simulink model "AttitudeComplementary"  (Simulink 6.6)
settings: Solver=ode4  StartTime=0.0  StopTime=300  FixedStep=SampleT  RelTol=1e-3
InitFcn:
  | clc
  | Taxi_Var_new
  | failures
  | insInit
values from neighbouring files (symbols this model uses):
  A1 = 0    [Taxi_Var.m]    (also in Taxi_Var_new.m = 0.007)
  Apolar = 0.0899    [Taxi_Var.m]    (also in Taxi_Var_new.m = 0.057)
  CD0 = 0.0219    [Taxi_Var.m]    (also in Taxi_Var_new.m = 0.022)
  chord = S/span    (= 0.384036716878)    [Taxi_Var.m]    (also in Taxi_Var_new.m = 0.351341681574)
  CL0 = 0.1857    [Taxi_Var.m]    (also in Taxi_Var_new.m = 0.38)
  CLa = 4.6206    [Taxi_Var.m]    (also in Taxi_Var_new.m = 18.5)
  CLa_dot = 1.93    [Taxi_Var.m]    (also in Taxi_Var_new.m = 2.64)
  Clb = -0.0043    [Taxi_Var.m]    (also in Taxi_Var_new.m = -0.06)
  ClDa = 0.1695    [Taxi_Var.m]    (also in Taxi_Var_new.m)
  CLDe = 0.4032    [Taxi_Var.m]    (also in Taxi_Var_new.m = 0.24)
  CLDf = 0.047    [Taxi_Var.m]    (also in Taxi_Var_new.m = 0.4)
  ClDr = 0.0003    [Taxi_Var.m]    (also in Taxi_Var_new.m = 0.055)
  Clp = -0.4425    [Taxi_Var.m]    (also in Taxi_Var_new.m = -0.88)
  CLq = 8.7465    [Taxi_Var.m]    (also in Taxi_Var_new.m = 7.4)
  Clr = 0.0675    [Taxi_Var.m]    (also in Taxi_Var_new.m = 0.04)
  Cm0 = -0.0902    [Taxi_Var.m]    (also in Taxi_Var_new.m = 0.56)
  Cma = -1.3995    [Taxi_Var.m]    (also in Taxi_Var_new.m = -1.58)
  CmDe = -0.9493    [Taxi_Var.m]    (also in Taxi_Var_new.m = -41)
  CmDf = -.021    (= -0.021)    [Taxi_Var.m]    (also in Taxi_Var_new.m)
  Cmq = -10.8760    (= -10.876)    [Taxi_Var.m]    (also in Taxi_Var_new.m = -12)
  Cnb = 0.0281    [Taxi_Var.m]    (also in Taxi_Var_new.m = 0.73)
  CnDa = -0.0031    [Taxi_Var.m]    (also in Taxi_Var_new.m = -0.032)
  CnDr = -0.0882    [Taxi_Var.m]    (also in Taxi_Var_new.m = 0.19)
  Cnp = -0.0695    [Taxi_Var.m]    (also in Taxi_Var_new.m = -0.1)
  Cnr = -0.1045    [Taxi_Var.m]    (also in Taxi_Var_new.m = -0.23)
  CYb = -0.1999    [Taxi_Var.m]    (also in Taxi_Var_new.m = -0.98)
  CYDr = 0.0192    [Taxi_Var.m]    (also in Taxi_Var_new.m = 0.066)
  Euler_0 = [0; 0; 45]'*pi/180    [Taxi_Var.m]    (also in Taxi_Var_new.m = [0 0 45]'*pi/180)
  ISA_g = 9.815    [Taxi_Var.m]    (also in Taxi_Var_new.m)
  Ixx = 3.689084    [Taxi_Var.m]    (also in Taxi_Var_new.m = 3.8)
  Iyy = 7.43789    [Taxi_Var.m]    (also in Taxi_Var_new.m = 9.58)
  Izz = 10.22202    [Taxi_Var.m]    (also in Taxi_Var_new.m = 9.68)
  mass = 22.5    [Taxi_Var.m]    (also in Taxi_Var_new.m = 8.16466266)
  MinThK = 0.075    [Taxi_Var.m]    (also in Taxi_Var_new.m = 0.077)
  Pos_0 = [0; 0; 1000]'    [Taxi_Var.m]    (also in Taxi_Var_new.m = [0 0 500]')
  PQR_0 = [0; 0; 0]'    [Taxi_Var.m]    (also in Taxi_Var_new.m = [ 0 0 0]'*pi/180)
  SampleT = 0.005    [failures.m]
  span = 2.3368    [Taxi_Var.m]    (also in Taxi_Var_new.m = 2.795)
  TFact = 0.4    [Taxi_Var.m]    (also in Taxi_Var_new.m)
  ThK = 2.18    [Taxi_Var.m]    (also in Taxi_Var_new.m = 2.17)
  Vb_0 = [35; 0; 0]'    [Taxi_Var.m]    (also in Taxi_Var_new.m = [35 0 0]')
undefined symbols (not defined in the file or in its folder): clock, DiscIntNeverNeededParam, Earth, gaind, polesd, sigbuilder_block, WGS84, zerosd
libraries: simulink x43, aerolibconvert2 x11, dspsigops x5, aerolibatmos2 x2, aerolibnav x2, dspmtrx3 x1, aerolibutil x1, aerolibtransform2 x1
(part 1 of 3)
CloseFcn:
  | rtwprivate ssgencode ModelCloseRequest AttitudeComplementary
settings Model: Creator=ASL_Lab  LastModifiedBy=ASL_Lab
settings DebuggingCC: MultiTaskDSMMsg=warning  MultiTaskCondExecSysMsg=none  StrictBusMsg=None
settings HardwareCC: TargetHWDeviceType=32-bit Generic
settings RTWCC: IncludeERTFirstTime=on

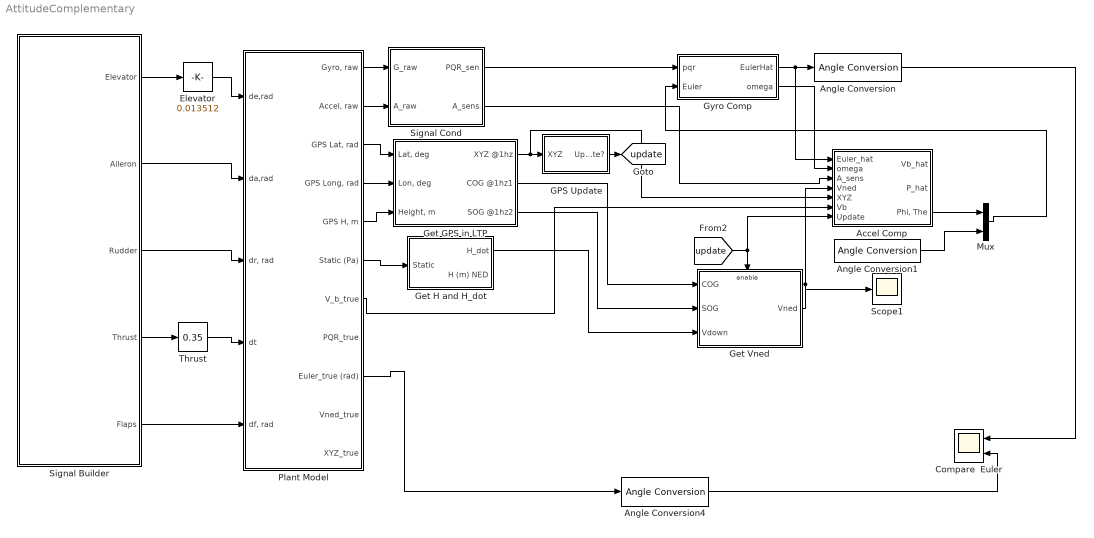
== system AttitudeComplementary ==
  Accel Comp : Subsystem
  Angle Conversion : aerolibconvert2/Angle Conversion  SystemSampleTime=-1  IU=rad  OU=deg
  Angle Conversion1 : aerolibconvert2/Angle Conversion  SystemSampleTime=-1  IU=deg  OU=rad
  Angle Conversion4 : aerolibconvert2/Angle Conversion  SystemSampleTime=-1  IU=rad  OU=deg
  Compare  Euler : Scope  NumInputPorts=2
      settings: TimeRange=150  YMin=-2.5~0  YMax=3.5~1.7  SaveName=ScopeData20
  Elevator : simulink/Math Operations/Slider Gain  SystemSampleTime=-1  low=-0.2  gain=0.013512  high=0.2
  GPS Update : Subsystem
  Get GPS in LTP : Subsystem
  "Get H and H_dot " : Subsystem
  Get Vned : Subsystem
  Gyro Comp : Subsystem
  Mux : Mux  Inputs=2
  Plant Model : Subsystem
  Scope1 : Scope
      settings: TimeRange=100  YMin=-60  YMax=80  SaveName=ScopeData27
  Signal Builder : Subsystem  Tag=STV Subsys  LoadFcn=sigbuilder_block('load');  StartFcn=sigbuilder_block('start');  StopFcn=sigbuilder_block('stop');  ClipboardFcn=sigbuilder_block('clipboard');  mask(Sigbuilder block){}
      mask help: Sigbuilder GUI
      mask init:
      | if ~strcmp(get_param(bdroot(gcbh),'SimulationStatus'),'stopped') tuvar = sigbuilder_block('maskInit'); end
      settings: CopyFcn=sigbuilder_block('copy');  DeleteFcn=sigbuilder_block('delete');  ModelCloseFcn=sigbuilder_block('modelClose');  PreSaveFcn=sigbuilder_block('preSave');  NameChangeFcn=sigbuilder_block('namechange');  OpenFcn=sigbuilder_block('open',[3 3 762 514.5 ]);  CloseFcn=sigbuilder_block('close');
      mask Display: plot(0,0,100,100,[10,10,40,40,10],[80,20,20,80,80],[40,10],[50,50], [40,27,10],[65,72,56],[40,25,25,10],[28,28,43,43]);
  Signal Cond : Subsystem
  Thrust : simulink/Math Operations/Slider Gain  SystemSampleTime=-1  low=0  gain=0.35  high=1
  tag scope: update=global
  wires:
  Signal Builder/4(Thrust) -> Thrust/1
  Thrust/1 -> Plant Model/4(dt)
  Signal Builder/1(Elevator) -> Elevator/1
  Signal Builder/2(Aileron) -> Plant Model/2(da,rad)
  Signal Builder/3(Rudder) -> Plant Model/3("dr, rad")
  Signal Builder/5(Flaps) -> Plant Model/5("df, rad")
  Elevator/1 -> Plant Model/1(de,rad)
  Plant Model/1("Gyro, raw") -> Signal Cond/1(G_raw)
  Plant Model/2("Accel, raw") -> Signal Cond/2(A_raw)
  Plant Model/3("GPS Lat, rad") -> Get GPS in LTP/1("Lat, deg")
  Plant Model/5("GPS H, m") -> Get GPS in LTP/3("Height, m")
  Plant Model/4("GPS Long, rad") -> Get GPS in LTP/2("Lon, deg")
  Signal Cond/2(A_sens) -> Accel Comp/3(A_sens)
  GPS Update/1(Update?) -> [update]
  Signal Cond/1(PQR_sen) -> Gyro Comp/1(pqr)
  [update] -> Get Vned/Enable, Accel Comp/7(Update)
  Gyro Comp/1(EulerHat) -> Angle Conversion/1, Accel Comp/1(Euler_hat)
  Angle Conversion/1 -> Compare  Euler/1
  Get Vned/1(Vned) -> Accel Comp/4(Vned), Scope1/1
  Accel Comp/3("Phi, The") -> Mux/1
  Angle Conversion1/1 -> Mux/2
  Mux/1 -> Gyro Comp/2(Euler)
  Plant Model/6(Static (Pa)) -> "Get H and H_dot "/1(Static)
  Get GPS in LTP/1(XYZ @1hz) -> GPS Update/1(XYZ), Accel Comp/5(XYZ)
  Gyro Comp/2(omega) -> Accel Comp/2(omega)
  Get GPS in LTP/2(COG @1hz1) -> Get Vned/1(COG)
  Get GPS in LTP/3(SOG @1hz2) -> Get Vned/2(SOG)
  "Get H and H_dot "/1(H_dot) -> Get Vned/3(Vdown)
  Plant Model/9(Euler_true (rad)) -> Angle Conversion4/1
  Plant Model/7(V_b_true) -> Accel Comp/6(Vb)
  Angle Conversion4/1 -> Compare  Euler/2

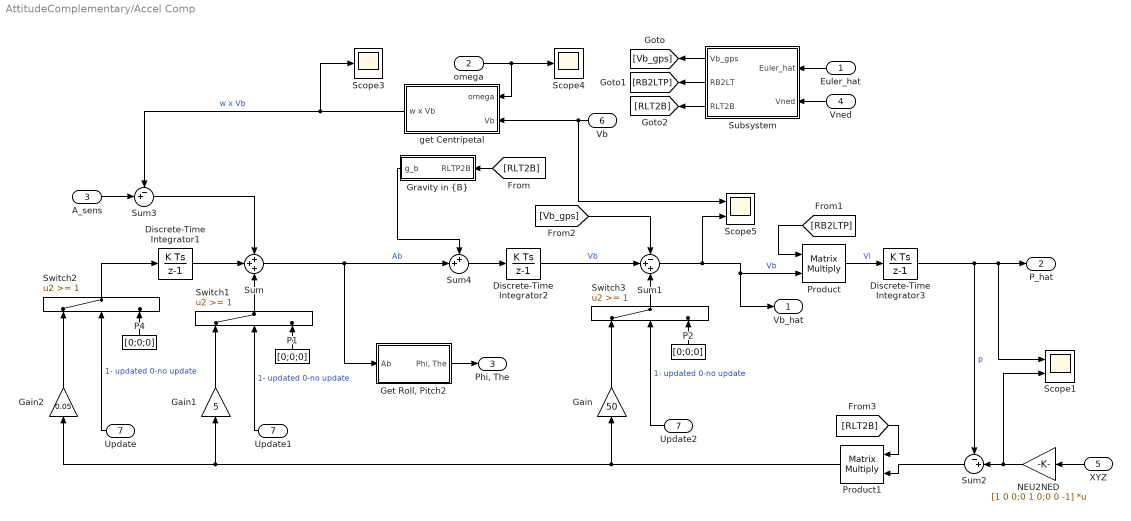
== system AttitudeComplementary/Accel Comp ==
  Euler_hat : Inport  Orientation=left
  omega : Inport  Port=2
  A_sens : Inport  Port=3
  Vned : Inport  Orientation=left  Port=4
  XYZ : Inport  Orientation=left  Port=5
  Vb : Inport  Orientation=left  Port=6
  Update : Inport  Orientation=left  Port=7
  Discrete-Time Integrator1 : DiscreteIntegrator  SampleTime=SampleT  ICPrevOutput=DiscIntNeverNeededParam  ICPrevScaledInput=DiscIntNeverNeededParam
  Discrete-Time Integrator2 : DiscreteIntegrator  InitialCondition=Vb_0  SampleTime=SampleT  ICPrevOutput=DiscIntNeverNeededParam  ICPrevScaledInput=DiscIntNeverNeededParam
  Discrete-Time Integrator3 : DiscreteIntegrator  InitialCondition=[Pos_0(1) Pos_0(2) -Pos_0(3)]  SampleTime=SampleT  ICPrevOutput=DiscIntNeverNeededParam  ICPrevScaledInput=DiscIntNeverNeededParam
  Gain : Gain  Orientation=up  Gain=50
  Gain1 : Gain  Orientation=up  Gain=5
  Gain2 : Gain  Orientation=up  Gain=0.05
  "Get Roll, Pitch2" : Subsystem
  "Gravity in {B}" : Subsystem  Orientation=left
  NEU2NED : Gain  Orientation=left  Gain=[1 0 0;0 1 0;0 0 -1]  Multiplication=Matrix(K*u)  SaturateOnIntegerOverflow=on
  P1 : Constant  Orientation=up  Value=[0;0;0]
  P2 : Constant  Orientation=up  Value=[0;0;0]
  P4 : Constant  Orientation=up  Value=[0;0;0]
  Product : Product  Multiplication=Matrix(*)  RndMeth=Zero
  Product1 : Product  Orientation=left  Multiplication=Matrix(*)  RndMeth=Zero
  Scope1 : Scope  NumInputPorts=2
      settings: TimeRange=300  YMin=-1500~-1500  YMax=8500~8500
  Scope3 : Scope
      settings: TimeRange=300  YMin=-10  YMax=4  SaveName=ScopeData26
  Scope4 : Scope
      settings: TimeRange=300  YMin=-0.1  YMax=0  SaveName=ScopeData29
  Scope5 : Scope  NumInputPorts=2
      settings: TimeRange=300  YMin=-2.5~-1750  YMax=35~3250  SaveName=ScopeData12
  Subsystem : Subsystem  Orientation=left
  Sum : Sum  Inputs=+++
  Sum1 : Sum  Inputs=-++
  Sum2 : Sum  Orientation=left  Inputs=-+|
  Sum3 : Sum  Inputs=-+|
  Sum4 : Sum  Inputs=++|
  Switch1 : Switch  Orientation=up  Threshold=1  SaturateOnIntegerOverflow=on
  Switch2 : Switch  Orientation=up  Threshold=1  SaturateOnIntegerOverflow=on
  Switch3 : Switch  Orientation=up  Threshold=1  SaturateOnIntegerOverflow=on
  Update1 : InportShadow  Orientation=left  Port=7  LatchByCopyingInsideSignal=off
  Update2 : InportShadow  Orientation=left  Port=7  LatchByCopyingInsideSignal=off
  get Centripetal : Subsystem  Orientation=left
  Vb_hat : Outport
  P_hat : Outport  Port=2
  "Phi, The" : Outport  Port=3
  wires:
  Sum2/1 -> Product1/2
  Discrete-Time Integrator3/1 -> Sum2/1, P_hat/1, Scope1/1  "p"
  Discrete-Time Integrator1/1 -> Sum/2
  Discrete-Time Integrator2/1 -> Sum1/2  "Vb"
  get Centripetal/1(w x Vb) -> Sum3/1, Scope3/1  "w x Vb"
  "Get Roll, Pitch2"/1("Phi, The") -> "Phi, The"/1
  A_sens/1 -> Sum3/2
  omega/1 -> get Centripetal/1(omega), Scope4/1
  Euler_hat/1 -> Subsystem/1(Euler_hat)
  Vned/1 -> Subsystem/2(Vned)
  Product/1 -> Discrete-Time Integrator3/1  "Vi"
  Sum1/1 -> Product/2, Vb_hat/1, Scope5/2  "Vb"
  XYZ/1 -> NEU2NED/1
  Subsystem/1(Vb_gps) -> [Vb_gps]
  Subsystem/2(RB2LT) -> [RB2LTP]
  Subsystem/3(RLT2B) -> [RLT2B]
  [RLT2B] -> "Gravity in {B}"/1(RLTP2B)
  [RB2LTP] -> Product/1
  NEU2NED/1 -> Sum2/2, Scope1/2
  [Vb_gps] -> Sum1/1
  [RLT2B] -> Product1/1
  Product1/1 -> Gain2/1, Gain1/1, Gain/1
  Vb/1 -> get Centripetal/2(Vb), Scope5/1
  P4/1 -> Switch2/3
  Update/1 -> Switch2/2  "1- updated 0-no update"
  Gain2/1 -> Switch2/1
  Switch2/1 -> Discrete-Time Integrator1/1
  P1/1 -> Switch1/3
  Update1/1 -> Switch1/2  "1- updated 0-no update"
  Switch1/1 -> Sum/3
  Gain1/1 -> Switch1/1
  P2/1 -> Switch3/3
  Update2/1 -> Switch3/2  "1- updated 0-no update"
  Gain/1 -> Switch3/1
  Switch3/1 -> Sum1/3
  Sum3/1 -> Sum/1
  Sum4/1 -> Discrete-Time Integrator2/1
  "Gravity in {B}"/1(g_b) -> Sum4/1
  Sum/1 -> Sum4/2, "Get Roll, Pitch2"/1(Ab)  "Ab"

== system AttitudeComplementary/GPS Update ==
  XYZ : Inport
  Demux : Demux  Outputs=3
  Detect Change : Subsystem
  Detect Change1 : Subsystem
  Detect Change2 : Subsystem
  Saturation1 : Saturate  UpperLimit=1  LowerLimit=0  SampleTime=SampleT
  Sum : Sum  Inputs=3
  Update? : Outport
  wires:
  Demux/1 -> Detect Change/1(Data)
  Demux/2 -> Detect Change1/1(Data)
  Demux/3 -> Detect Change2/1(Data)
  Detect Change/1(change?) -> Sum/1
  Detect Change1/1(change?) -> Sum/2
  Detect Change2/1(change?) -> Sum/3
  Sum/1 -> Saturation1/1
  XYZ/1 -> Demux/1
  Saturation1/1 -> Update?/1

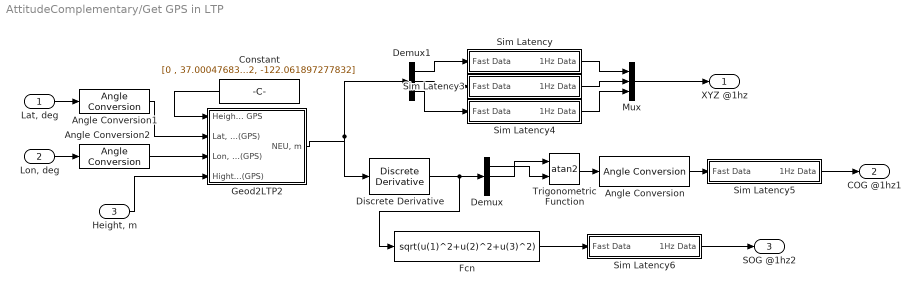
== system AttitudeComplementary/Get GPS in LTP ==
  "Lat, deg" : Inport
  "Lon, deg" : Inport  Port=2
  "Height, m" : Inport  Port=3
  Angle Conversion : aerolibconvert2/Angle Conversion  SystemSampleTime=-1  IU=rad  OU=deg
  Angle Conversion1 : aerolibconvert2/Angle Conversion  SystemSampleTime=-1  IU=rad  OU=deg
  Angle Conversion2 : aerolibconvert2/Angle Conversion  SystemSampleTime=-1  IU=rad  OU=deg
  Constant : Constant  Orientation=left  Value=[0 , 37.0004768371582, -122.061897277832]
  Demux : Demux  Outputs=3
  Demux1 : Demux  Outputs=3
  Discrete Derivative : simulink/Discrete/Discrete Derivative  SystemSampleTime=-1  gainval=1.0  ICPrevScaledInput=0.0  OutDataType=sfix(16)  OutScaling=2^-10  DoSatur=off
  Fcn : Fcn  Expr=sqrt(u(1)^2+u(2)^2+u(3)^2)
  Geod2LTP2 : Subsystem
      mask Description:
      | This block provides transformation of the Geodetic coordinates
      | to the LTP coorinate system. The block uses two consecutive transformations
      | (Geodetic -> ECEF ->LTP).
      | Geodetic coordinates of the LTP origin should also be predetermined.
      mask Help: Oops!
      mask Display: plot(0,0,100,100,[45,40,35,40,40],[85,95,85,95,40],[85,95,85,95,40],[35,40,45,40,40],[60,40,10,20,10,14],[70,40,10,13,10,20],[56,45],[70,70],[60,60],[50,60],[60,60],[30,40],[50,60],[20,20],[30,40],[20,20],[45,55],[35,25],[75,65],[35,25])
  Mux : Mux  Inputs=3
  Sim Latency : Subsystem
  Sim Latency3 : Subsystem
  Sim Latency4 : Subsystem
  Sim Latency5 : Subsystem
  Sim Latency6 : Subsystem
  Trigonometric Function : Trigonometry  Operator=atan2
  XYZ @1hz : Outport
  COG @1hz1 : Outport  Port=2
  SOG @1hz2 : Outport  Port=3
  wires:
  Constant/1 -> Geod2LTP2/1("Height, Lat, Lon Initials from GPS")
  Geod2LTP2/1("NEU, m") -> Discrete Derivative/1, Demux1/1
  "Lat, deg"/1 -> Angle Conversion1/1
  "Lon, deg"/1 -> Angle Conversion2/1
  "Height, m"/1 -> Geod2LTP2/4(Hight,m(GPS))
  Fcn/1 -> Sim Latency6/1(Fast Data)
  Demux/2 -> Trigonometric Function/1
  Demux/1 -> Trigonometric Function/2
  Trigonometric Function/1 -> Angle Conversion/1
  Angle Conversion/1 -> Sim Latency5/1(Fast Data)
  Discrete Derivative/1 -> Demux/1, Fcn/1
  Mux/1 -> XYZ @1hz/1
  Angle Conversion1/1 -> Geod2LTP2/2("Lat, deg(GPS)")
  Angle Conversion2/1 -> Geod2LTP2/3("Lon, deg(GPS)")
  Demux1/1 -> Sim Latency/1(Fast Data)
  Demux1/2 -> Sim Latency3/1(Fast Data)
  Demux1/3 -> Sim Latency4/1(Fast Data)
  Sim Latency/1(1Hz Data) -> Mux/1
  Sim Latency3/1(1Hz Data) -> Mux/2
  Sim Latency4/1(1Hz Data) -> Mux/3
  Sim Latency5/1(1Hz Data) -> COG @1hz1/1
  Sim Latency6/1(1Hz Data) -> SOG @1hz2/1

== system AttitudeComplementary/Get H and H_dot  ==
  Static : Inport
  Discrete Derivative : simulink/Discrete/Discrete Derivative  SystemSampleTime=-1  gainval=1.0  ICPrevScaledInput=0.0  OutDataType=sfix(16)  OutScaling=2^-10  DoSatur=off
  Gain : Gain  Gain=-1
  Pressure Altitude : aerolibatmos2/Pressure Altitude  SystemSampleTime=-1  units=Metric (MKS)  action=Warning
  H_dot : Outport
  H (m) NED : Outport  Port=2
  wires:
  Pressure Altitude/1 -> Gain/1
  Gain/1 -> Discrete Derivative/1, H (m) NED/1
  Discrete Derivative/1 -> H_dot/1
  Static/1 -> Pressure Altitude/1

== system AttitudeComplementary/Get Vned ==
  COG : Inport
  SOG : Inport  Port=2
  Vdown : Inport  Port=3
  Enable : EnablePort
  Embedded MATLAB Function1 : Stateflow chart
  Mux1 : Mux  Inputs=3
  Vned : Outport
  wires:
  Embedded MATLAB Function1/1(Vn) -> Mux1/1
  Embedded MATLAB Function1/2(Ve) -> Mux1/2
  Vdown/1 -> Mux1/3
  Mux1/1 -> Vned/1
  COG/1 -> Embedded MATLAB Function1/2(cog)
  SOG/1 -> Embedded MATLAB Function1/1(sog)

== system AttitudeComplementary/Gyro Comp ==
  pqr : Inport
  Euler : Inport  Orientation=left  Port=2
  Constant : Constant  Value=[1 0 0]
  Discrete-Time Integrator1 : DiscreteIntegrator  SampleTime=SampleT  ICPrevOutput=DiscIntNeverNeededParam  ICPrevScaledInput=DiscIntNeverNeededParam
  Discrete-Time Integrator2 : DiscreteIntegrator  InitialCondition=PQR_0  SampleTime=SampleT  ICPrevOutput=DiscIntNeverNeededParam  ICPrevScaledInput=DiscIntNeverNeededParam
  Discrete-Time Integrator3 : DiscreteIntegrator  InitialCondition=Euler_0  SampleTime=SampleT  ICPrevOutput=DiscIntNeverNeededParam  ICPrevScaledInput=DiscIntNeverNeededParam
  Embedded MATLAB Function : Stateflow chart
  Gain : Gain  Orientation=up  Gain=3
  Gain1 : Gain  Orientation=up  Gain=0.5
  Gain2 : Gain  Orientation=up  Gain=0.01
  Integer Delay : simulink/Discrete/Integer Delay  Orientation=left  vinit=0.0  samptime=-1  NumDelays=1
  Scope : Scope
      settings: YMin=-0.08  YMax=0.035  SaveName=ScopeData4
  Scope1 : Scope
      settings: YMin=-0.08  YMax=0.035  SaveName=ScopeData28
  Slider Gain : simulink/Math Operations/Slider Gain  SystemSampleTime=-1  low=0  gain=0.01  high=0.09
  Sum : Sum  Inputs=+++
  Sum1 : Sum  Inputs=|++
  Sum2 : Sum  Orientation=left  Inputs=-+|
  Sum3 : Sum  Inputs=|++
  EulerHat : Outport
  omega : Outport  Port=2
  wires:
  Discrete-Time Integrator2/1 -> Sum/2
  Sum1/1 -> Discrete-Time Integrator2/1
  Discrete-Time Integrator1/1 -> Sum1/1, Scope1/1
  Gain/1 -> Sum/3
  Gain1/1 -> Sum1/2
  Gain2/1 -> Discrete-Time Integrator1/1
  Discrete-Time Integrator3/1 -> EulerHat/1, Sum2/1, Integer Delay/1, Scope/1
  Euler/1 -> Sum2/2
  Sum2/1 -> Gain2/1, Gain1/1, Gain/1
  Sum/1 -> omega/1, Embedded MATLAB Function/2(pqr)
  Embedded MATLAB Function/1(lamDot) -> Discrete-Time Integrator3/1
  Integer Delay/1 -> Embedded MATLAB Function/1(lam)
  pqr/1 -> Sum3/1
  Sum3/1 -> Sum/1
  Constant/1 -> Slider Gain/1
  Slider Gain/1 -> Sum3/2

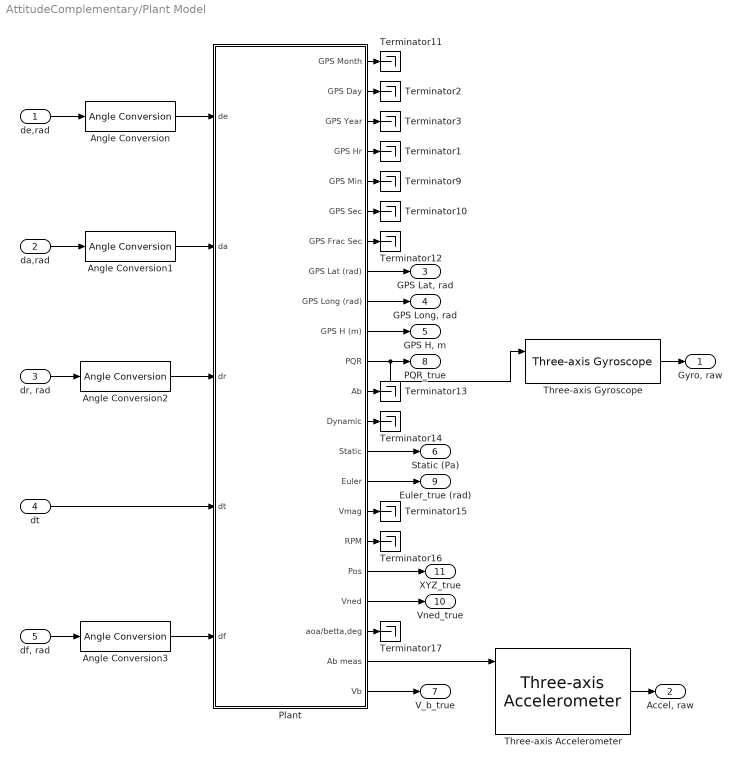
== system AttitudeComplementary/Plant Model ==
  de,rad : Inport
  da,rad : Inport  Port=2
  "dr, rad" : Inport  Port=3
  dt : Inport  Port=4
  "df, rad" : Inport  Port=5
  Angle Conversion{,1..3} (4 alike) : aerolibconvert2/Angle Conversion  SystemSampleTime=-1  IU=rad  OU=deg
  Plant : Subsystem
  Terminator{1..3,9..17} (12 alike) : Terminator
  Three-axis Accelerometer : aerolibnav/Three-axis Accelerometer  SystemSampleTime=-1  units=Metric (MKS)  acc=[0 0 0]  gtype=off  dtype_a=on  w_a=190  z_a=0.707  a_sf_cc=[-41 0 0; 0 41 0; 0 0 -43]  a_bias=[2015 2018 2006]  a_rand=on  a_seeds=[23093 23094 23095]  a_pow=[0.008 0.008 0.008]  a_sat="[-inf  -inf  -inf  inf inf inf]"  a_Ts=SampleT
  Three-axis Gyroscope : aerolibnav/Three-axis Gyroscope  SystemSampleTime=-1  dtype_g=on  w_g=190  z_g=0.707  g_sf_cc=[-142 0 0; 0 142 0; 0 0 235]  g_bias=[1866 1981 2042]  g_sen=[0 0 0]  g_rand=on  g_seeds=[23093 23094 23095]  g_pow=[0.008 0.008 0.008]  g_sat="[-inf  -inf  -inf  inf inf inf]"  g_Ts=SampleT
  "Gyro, raw" : Outport
  "Accel, raw" : Outport  Port=2
  "GPS Lat, rad" : Outport  Port=3
  "GPS Long, rad" : Outport  Port=4
  "GPS H, m" : Outport  Port=5
  Static (Pa) : Outport  Port=6
  V_b_true : Outport  Port=7
  PQR_true : Outport  Port=8
  Euler_true (rad) : Outport  Port=9
  Vned_true : Outport  Port=10
  XYZ_true : Outport  Port=11
  wires:
  Three-axis Gyroscope/1 -> "Gyro, raw"/1
  Three-axis Accelerometer/1 -> "Accel, raw"/1
  Plant/11(PQR) -> PQR_true/1, Three-axis Gyroscope/1
  Plant/14(Static) -> Static (Pa)/1
  Plant/8(GPS Lat (rad)) -> "GPS Lat, rad"/1
  Plant/9(GPS Long (rad)) -> "GPS Long, rad"/1
  Plant/10(GPS H (m)) -> "GPS H, m"/1
  Plant/21(Ab meas) -> Three-axis Accelerometer/1
  Plant/22(Vb) -> V_b_true/1
  Plant/15(Euler) -> Euler_true (rad)/1
  Plant/19(Vned) -> Vned_true/1
  Plant/18(Pos) -> XYZ_true/1
  Plant/1(GPS Month) -> Terminator11/1
  Plant/2(GPS Day) -> Terminator2/1
  Plant/3(GPS Year) -> Terminator3/1
  Plant/4(GPS Hr) -> Terminator1/1
  Plant/5(GPS Min) -> Terminator9/1
  Plant/6(GPS Sec) -> Terminator10/1
  Plant/7(GPS Frac Sec) -> Terminator12/1
  Plant/12(Ab) -> Terminator13/1
  Plant/13(Dynamic) -> Terminator14/1
  Plant/16(Vmag) -> Terminator15/1
  Plant/17(RPM) -> Terminator16/1
  Plant/20(aoa/betta,deg) -> Terminator17/1
  de,rad/1 -> Angle Conversion/1
  da,rad/1 -> Angle Conversion1/1
  "dr, rad"/1 -> Angle Conversion2/1
  dt/1 -> Plant/4(dt)
  "df, rad"/1 -> Angle Conversion3/1
  Angle Conversion/1 -> Plant/1(de)
  Angle Conversion1/1 -> Plant/2(da)
  Angle Conversion2/1 -> Plant/3(dr)
  Angle Conversion3/1 -> Plant/5(df)

== system AttitudeComplementary/Signal Builder ==
  Demux : Demux  Tag=STV Demux  Outputs=5
  FromWs : FromWorkspace  Tag=STV FromWs  VariableName=tuvar  SampleTime=0  SigBuilderData=DataTag0  VnvData=DataTag1
      SigBuilderData=|
      | channels(1).label = 'Elevator'
      | channels(1).allXData = {[0 200], [0 200], [0 100 100 200]}
      | channels(1).allYData = {[0.2 0.2], [1 1], [-0.07 -0.07 0 -0.07]}
      | channels(2).label = 'Aileron'
      | channels(2).allXData = {[0 80 80.01 84 84.01 88 88.01 200], [0 200], [0 200]}
      | channels(2).allYData = {[0 0 3 3 -3 -3 0 0], [0 0], [0 0]}
      | channels(3).label = 'Rudder'
      | channels(3).allXData = {[0 200], [0 200], [0 200]}
      | channels(3).allYData = {[0 0], [0 0], [0 0]}
      | channels(4).label = 'Thrust'
      | channels(4).allXData = {[0 200], [0 200], [0 200]}
      | channels(4).allYData = {[0.125 0.125], [1 1], [1 1]}
      | channels(5).label = 'Flaps'
      | channels(5).allXData = {[0 200], [0 200], [0 200]}
      | channels(5).allYData = {[0 0], [0 0], [0 0]}
      | common.afterFinalStr = 'Extrapolate'
      | common.sampleTime = 0
      | dataSet(1).timeRange = [0 200]
      | dataSet(1).name = 'Aileron 5 Deg'
      | dataSet(2).timeRange = [0 200]
      | dataSet(2).name = 'Trim'
      | dataSet(3).timeRange = [0 200]
      | dataSet(3).name = 'Elevator'
  Elevator : Outport  Tag=STV Outport
  Aileron : Outport  Tag=STV Outport  Port=2
  Rudder : Outport  Tag=STV Outport  Port=3
  Thrust : Outport  Tag=STV Outport  Port=4
  Flaps : Outport  Tag=STV Outport  Port=5
  wires:
  Demux/1 -> Elevator/1
  FromWs/1 -> Demux/1
  Demux/2 -> Aileron/1
  Demux/3 -> Rudder/1
  Demux/4 -> Thrust/1
  Demux/5 -> Flaps/1

== system AttitudeComplementary/Signal Cond ==
  G_raw : Inport
  A_raw : Inport  Port=2
  Accel Convert : Subsystem
  Gyro Convert : Subsystem
  PQR_sen : Outport
  A_sens : Outport  Port=2
  wires:
  G_raw/1 -> Gyro Convert/1(Raw)
  Gyro Convert/1(Comp) -> PQR_sen/1
  A_raw/1 -> Accel Convert/1(Raw)
  Accel Convert/1(Comp) -> A_sens/1

== system AttitudeComplementary/Accel Comp/Get Roll, Pitch2 ==
  Ab : Inport
  Fcn : Fcn  Expr=atan2(u(1),-u(3))
  Fcn1 : Fcn  Expr=atan2(u(2),-u(3))
  Mux : Mux  Inputs=2
  "Phi, The" : Outport
  wires:
  Fcn1/1 -> Mux/1
  Fcn/1 -> Mux/2
  Ab/1 -> Fcn1/1, Fcn/1
  Mux/1 -> "Phi, The"/1

== system AttitudeComplementary/Accel Comp/Gravity in {B} ==
  RLTP2B : Inport  Orientation=left
  "Gravity {I}" : Constant  Orientation=left  Value=[0 0 ISA_g]
  Product1 : Product  Orientation=left  Multiplication=Matrix(*)  RndMeth=Zero
  g_b : Outport  Orientation=left
  wires:
  "Gravity {I}"/1 -> Product1/2
  RLTP2B/1 -> Product1/1
  Product1/1 -> g_b/1

== system AttitudeComplementary/Accel Comp/Subsystem ==
  Euler_hat : Inport  Orientation=left
  Vned : Inport  Orientation=left  Port=2
  Integer Delay2 : simulink/Discrete/Integer Delay  Orientation=left  vinit=0.0  samptime=-1  NumDelays=1
  LTP2B : dspmtrx3/Transpose  Orientation=left  SystemSampleTime=-1  Hermitian=off  overflowFlag=off
  Product : Product  Orientation=left  Multiplication=Matrix(*)  RndMeth=Zero
  RB2LTP : Subsystem  Orientation=left
  Vb_gps : Outport  Orientation=left
  RB2LT : Outport  Orientation=left  Port=2
  RLT2B : Outport  Orientation=left  Port=3
  wires:
  Euler_hat/1 -> Integer Delay2/1
  Integer Delay2/1 -> RB2LTP/1(Euler)
  LTP2B/1 -> Product/1, RLT2B/1
  Vned/1 -> Product/2
  RB2LTP/1(Rot) -> LTP2B/1, RB2LT/1
  Product/1 -> Vb_gps/1

== system AttitudeComplementary/Accel Comp/get Centripetal ==
  omega : Inport  Orientation=left
  Vb : Inport  Orientation=left  Port=2
  3vector LPF : Subsystem  Orientation=left  mask{flpf=0.3}
      mask prompts: flpf "LowPass Freq"
      mask Display: droots([],-flpf,flpf)
  3x3 Cross Product : aerolibutil/3x3 Cross Product  Orientation=left  SystemSampleTime=-1
  Integer Delay : simulink/Discrete/Integer Delay  Orientation=left  vinit=0.0  samptime=-1  NumDelays=1
  Integer Delay1 : simulink/Discrete/Integer Delay  Orientation=left  vinit=0.0  samptime=-1  NumDelays=1
  w x Vb : Outport  Orientation=left
  wires:
  Integer Delay1/1 -> 3x3 Cross Product/1
  Integer Delay/1 -> 3x3 Cross Product/2
  omega/1 -> 3vector LPF/1(In1)
  Vb/1 -> Integer Delay/1
  3x3 Cross Product/1 -> w x Vb/1  "w x Vb"
  3vector LPF/1(Out1) -> Integer Delay1/1

== system AttitudeComplementary/GPS Update/Detect Change ==
  Data : Inport
  Abs1 : Abs
  Difference1 : simulink/Discrete/Difference  SystemSampleTime=-1  ICPrevInput=0.0  OutDataType=sfix(16)  OutScaling=2^-10  DoSatur=off
  Saturation1 : Saturate  UpperLimit=1  LowerLimit=0  SampleTime=SampleT
  change? : Outport
  wires:
  Difference1/1 -> Abs1/1
  Abs1/1 -> Saturation1/1
  Data/1 -> Difference1/1
  Saturation1/1 -> change?/1

== system AttitudeComplementary/GPS Update/Detect Change1 ==
  Data : Inport
  Abs1 : Abs
  Difference1 : simulink/Discrete/Difference  SystemSampleTime=-1  ICPrevInput=0.0  OutDataType=sfix(16)  OutScaling=2^-10  DoSatur=off
  Saturation1 : Saturate  UpperLimit=1  LowerLimit=0  SampleTime=SampleT
  change? : Outport
  wires:
  Saturation1/1 -> change?/1
  Data/1 -> Difference1/1
  Abs1/1 -> Saturation1/1
  Difference1/1 -> Abs1/1

== system AttitudeComplementary/GPS Update/Detect Change2 ==
  Data : Inport
  Abs1 : Abs
  Difference1 : simulink/Discrete/Difference  SystemSampleTime=-1  ICPrevInput=0.0  OutDataType=sfix(16)  OutScaling=2^-10  DoSatur=off
  Saturation1 : Saturate  UpperLimit=1  LowerLimit=0  SampleTime=SampleT
  change? : Outport
  wires:
  Difference1/1 -> Abs1/1
  Abs1/1 -> Saturation1/1
  Data/1 -> Difference1/1
  Saturation1/1 -> change?/1

== system AttitudeComplementary/Get GPS in LTP/Geod2LTP2 ==
  "Height, Lat, Lon Initials from GPS" : Inport
  "Lat, deg(GPS)" : Inport  Port=2
  "Lon, deg(GPS)" : Inport  Port=3
  Hight,m(GPS) : Inport  Port=4
  Demux : Demux  Outputs=3
  ECEF2LTP (UEN) : Subsystem
      mask Display: plot(0,0,100,100,[45,40,35,40,40],[85,95,85,95,40],[85,95,85,95,40],[35,40,45,40,40],[60,40,10,20,10,14],[70,40,10,13,10,20],[56,45],[70,70],[60,60],[50,60],[60,60],[30,40],[50,60],[20,20],[30,40],[20,20],[45,55],[35,25],[75,65],[35,25])
  Geod2ECEF : Subsystem  mask{Re=6378137, Rp=6356752.3142}
      mask prompts: Re "Enter equatorial radius, m"; Rp "Enter polar radius,m"
  Geod2ECEF1 : Subsystem  mask{Re=6378137, Rp=6356752.3142}
      mask prompts: Re "Enter equatorial radius, m"; Rp "Enter polar radius,m"
  Mux : Mux  Inputs=3
  Mux1 : Mux  Inputs=2
  Mux2 : Mux  Inputs=3
  Reshape : Reshape  OutputDimensionality=Column vector (2-D)
  Sum1 : Sum  Inputs=|+-  SaturateOnIntegerOverflow=on
  UEN 2 NEU : Gain  Gain=[0 0 1;0 1 0;1 0 0]  Multiplication=Matrix(K*u)  SaturateOnIntegerOverflow=on
  "NEU, m" : Outport
  wires:
  UEN 2 NEU/1 -> "NEU, m"/1
  Geod2ECEF/3("Ze, m ") -> Mux/3
  Geod2ECEF/1("Xe, m ") -> Mux/1
  Geod2ECEF/2("Ye, m ") -> Mux/2
  "Lat, deg(GPS)"/1 -> Geod2ECEF/2("lat, deg")
  "Lon, deg(GPS)"/1 -> Geod2ECEF/3(lon,deg)
  Mux1/1 -> ECEF2LTP (UEN)/2("Long, Lat")
  Geod2ECEF1/3("Ze, m ") -> Mux2/3
  Geod2ECEF1/1("Xe, m ") -> Mux2/1
  Geod2ECEF1/2("Ye, m ") -> Mux2/2
  Mux2/1 -> Sum1/2  "R_in"
  Demux/1 -> Geod2ECEF1/1("height, m")
  Demux/2 -> Mux1/2, Geod2ECEF1/2("lat, deg")
  Demux/3 -> Mux1/1, Geod2ECEF1/3(lon,deg)
  ECEF2LTP (UEN)/1(Out) -> Reshape/1  "Moving Side"
  Hight,m(GPS)/1 -> Geod2ECEF/1("height, m")
  "Height, Lat, Lon Initials from GPS"/1 -> Demux/1
  Mux/1 -> Sum1/1  "r_mov"
  Sum1/1 -> ECEF2LTP (UEN)/1(ECEF coordinates)
  Reshape/1 -> UEN 2 NEU/1

== system AttitudeComplementary/Get GPS in LTP/Sim Latency ==
  Fast Data : Inport
  Counter Free-Running1 : simulink/Sources/Counter Free-Running  SystemSampleTime=-1  NumBits=1  tsamp=1
  Rate Transition2 : RateTransition  OutPortSampleTime=SampleT
  Sample and Hold : dspsigops/Sample and Hold  SystemSampleTime=-1  trig=Either edge  initCond=0  latchinput=off
  1Hz Data : Outport
  wires:
  Sample and Hold/1 -> 1Hz Data/1
  Fast Data/1 -> Sample and Hold/1
  Rate Transition2/1 -> Sample and Hold/Trigger
  Counter Free-Running1/1 -> Rate Transition2/1

== system AttitudeComplementary/Get GPS in LTP/Sim Latency3 ==
  Fast Data : Inport
  Counter Free-Running1 : simulink/Sources/Counter Free-Running  SystemSampleTime=-1  NumBits=1  tsamp=1
  Rate Transition2 : RateTransition  OutPortSampleTime=SampleT
  Sample and Hold : dspsigops/Sample and Hold  SystemSampleTime=-1  trig=Either edge  initCond=0  latchinput=off
  1Hz Data : Outport
  wires:
  Counter Free-Running1/1 -> Rate Transition2/1
  Rate Transition2/1 -> Sample and Hold/Trigger
  Fast Data/1 -> Sample and Hold/1
  Sample and Hold/1 -> 1Hz Data/1

== system AttitudeComplementary/Get GPS in LTP/Sim Latency4 ==
  Fast Data : Inport
  Counter Free-Running1 : simulink/Sources/Counter Free-Running  SystemSampleTime=-1  NumBits=1  tsamp=1
  Rate Transition2 : RateTransition  OutPortSampleTime=SampleT
  Sample and Hold : dspsigops/Sample and Hold  SystemSampleTime=-1  trig=Either edge  initCond=0  latchinput=off
  1Hz Data : Outport
  wires:
  Sample and Hold/1 -> 1Hz Data/1
  Fast Data/1 -> Sample and Hold/1
  Rate Transition2/1 -> Sample and Hold/Trigger
  Counter Free-Running1/1 -> Rate Transition2/1

== system AttitudeComplementary/Get GPS in LTP/Sim Latency5 ==
  Fast Data : Inport
  Counter Free-Running1 : simulink/Sources/Counter Free-Running  SystemSampleTime=-1  NumBits=1  tsamp=1
  Rate Transition2 : RateTransition  OutPortSampleTime=SampleT
  Sample and Hold : dspsigops/Sample and Hold  SystemSampleTime=-1  trig=Either edge  initCond=0  latchinput=off
  1Hz Data : Outport
  wires:
  Counter Free-Running1/1 -> Rate Transition2/1
  Rate Transition2/1 -> Sample and Hold/Trigger
  Fast Data/1 -> Sample and Hold/1
  Sample and Hold/1 -> 1Hz Data/1

== system AttitudeComplementary/Get GPS in LTP/Sim Latency6 ==
  Fast Data : Inport
  Counter Free-Running1 : simulink/Sources/Counter Free-Running  SystemSampleTime=-1  NumBits=1  tsamp=1
  Rate Transition2 : RateTransition  OutPortSampleTime=SampleT
  Sample and Hold : dspsigops/Sample and Hold  SystemSampleTime=-1  trig=Either edge  initCond=0  latchinput=off
  1Hz Data : Outport
  wires:
  Sample and Hold/1 -> 1Hz Data/1
  Fast Data/1 -> Sample and Hold/1
  Rate Transition2/1 -> Sample and Hold/Trigger
  Counter Free-Running1/1 -> Rate Transition2/1

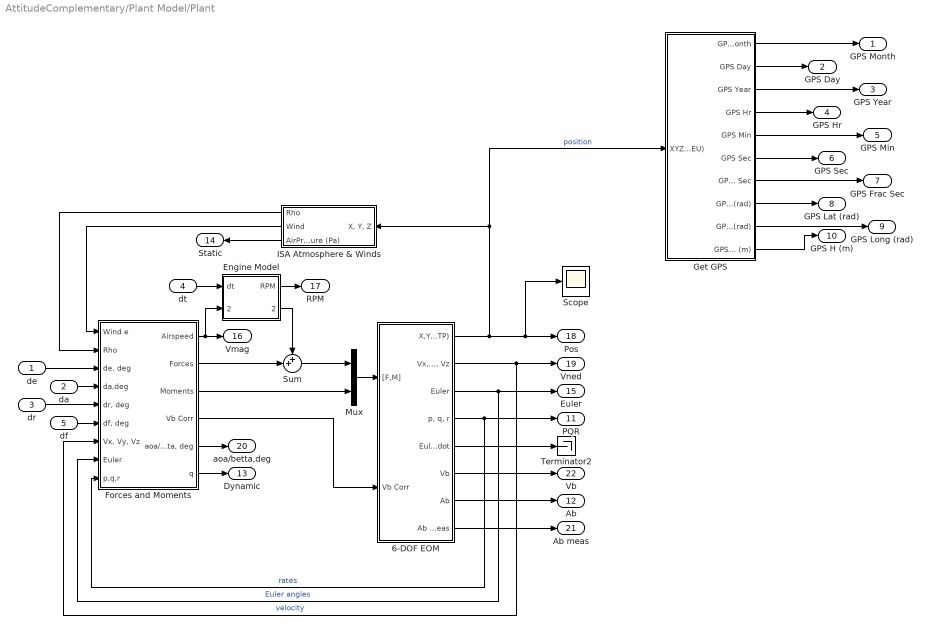
== system AttitudeComplementary/Plant Model/Plant ==
  de : Inport
  da : Inport  Port=2
  dr : Inport  Port=3
  dt : Inport  Port=4
  df : Inport  Port=5
  6-DOF EOM : Subsystem
  Engine Model : Subsystem
  Forces and Moments : Subsystem
  Get GPS : Subsystem
  ISA Atmosphere & Winds : Subsystem  Orientation=left
  Mux : Mux  Inputs=2
  Scope : Scope
      settings: YMin=0  YMax=5250
  Sum : Sum  Inputs=++|  SaturateOnIntegerOverflow=on
  Terminator2 : Terminator
  GPS Month : Outport
  GPS Day : Outport  Port=2
  GPS Year : Outport  Port=3
  GPS Hr : Outport  Port=4
  GPS Min : Outport  Port=5
  GPS Sec : Outport  Port=6
  GPS Frac Sec : Outport  Port=7
  GPS Lat (rad) : Outport  Port=8
  GPS Long (rad) : Outport  Port=9
  GPS H (m) : Outport  Port=10
  PQR : Outport  Port=11
  Ab : Outport  Port=12
  Dynamic : Outport  Port=13
  Static : Outport  Orientation=left  Port=14
  Euler : Outport  Port=15
  Vmag : Outport  Port=16
  RPM : Outport  Port=17
  Pos : Outport  Port=18
  Vned : Outport  Port=19
  aoa/betta,deg : Outport  Port=20
  Ab meas : Outport  Port=21
  Vb : Outport  Port=22
  wires:
  Get GPS/1(GPS Month) -> GPS Month/1
  Get GPS/2(GPS Day) -> GPS Day/1
  Get GPS/3(GPS Year) -> GPS Year/1
  Get GPS/4(GPS Hr) -> GPS Hr/1
  Get GPS/5(GPS Min) -> GPS Min/1
  Get GPS/6(GPS Sec) -> GPS Sec/1
  Get GPS/7(GPS Frac Sec) -> GPS Frac Sec/1
  Get GPS/8(GPS Lat (rad)) -> GPS Lat (rad)/1
  Get GPS/9(GPS Long (rad)) -> GPS Long (rad)/1
  Get GPS/10(GPS H (m)) -> GPS H (m)/1
  6-DOF EOM/8(Ab meas) -> Ab meas/1
  Mux/1 -> 6-DOF EOM/1("[F,M]")
  6-DOF EOM/5(Euler_dot) -> Terminator2/1
  6-DOF EOM/6(Vb) -> Vb/1
  Engine Model/1(RPM) -> RPM/1
  Engine Model/2(Thrust) -> Sum/1
  Forces and Moments/6(q) -> Dynamic/1
  ISA Atmosphere & Winds/3(AirPressure (Pa)) -> Static/1
  Forces and Moments/1(Airspeed) -> Engine Model/2(Vmag), Vmag/1
  ISA Atmosphere & Winds/2(Wind) -> Forces and Moments/1(Wind e)
  ISA Atmosphere & Winds/1(Rho) -> Forces and Moments/2(Rho)
  Forces and Moments/3(Moments) -> Mux/2
  Forces and Moments/2(Forces) -> Sum/2
  Sum/1 -> Mux/1
  Forces and Moments/4(Vb Corr) -> 6-DOF EOM/2(Vb Corr)
  6-DOF EOM/1(X,Y,Z (LTP)) -> ISA Atmosphere & Winds/1("X, Y, Z"), Get GPS/1(XYZ (NEU)), Pos/1, Scope/1  "position"
  6-DOF EOM/2("Vx, Vy, Vz") -> Vned/1, Forces and Moments/7("Vx, Vy, Vz ")  "velocity"
  6-DOF EOM/3(Euler) -> Forces and Moments/8(Euler), Euler/1  "Euler angles"
  6-DOF EOM/4("p, q, r") -> PQR/1, Forces and Moments/9(p,q,r)  "rates"
  6-DOF EOM/7(Ab) -> Ab/1
  Forces and Moments/5("aoa/betta, deg") -> aoa/betta,deg/1
  dt/1 -> Engine Model/1(dt)
  de/1 -> Forces and Moments/3("de, deg")
  da/1 -> Forces and Moments/4(da,deg)
  dr/1 -> Forces and Moments/5("dr, deg")
  df/1 -> Forces and Moments/6("df, deg")

== system AttitudeComplementary/Signal Cond/Accel Convert ==
  Raw : Inport
  3vector LPF : Subsystem  mask{flpf=5}
      mask prompts: flpf "LowPass Freq"
      mask Display: droots([],-flpf,flpf)
  Bias : Constant  Value=[2015 2018 2006]
  Divide : Product  Inputs=/*  OutScaling=2^-10
  Gains : Constant  Value=[-41 41 -43]
  Scope2 : Scope
      settings: TimeRange=100  YMin=-14.06123404388128  YMax=1.094597546893038  SaveName=ScopeData25
  Sum : Sum  Inputs=|+-
  Comp : Outport
  wires:
  Raw/1 -> 3vector LPF/1(In1)
  Divide/1 -> Comp/1, Scope2/1
  Sum/1 -> Divide/2
  Gains/1 -> Divide/1
  Bias/1 -> Sum/2
  3vector LPF/1(Out1) -> Sum/1

== system AttitudeComplementary/Signal Cond/Gyro Convert ==
  Raw : Inport
  3vector LPF : Subsystem  mask{flpf=5}
      mask prompts: flpf "LowPass Freq"
      mask Display: droots([],-flpf,flpf)
  Bias : Constant  Value=[1866 1981 2042]
  Divide : Product  Inputs=/*  OutScaling=2^-10
  Gains : Constant  Value=[-142 142 235]
  Sum : Sum  Inputs=|+-
  Comp : Outport
  wires:
  Bias/1 -> Sum/2
  Gains/1 -> Divide/1
  Sum/1 -> Divide/2
  Divide/1 -> Comp/1
  Raw/1 -> 3vector LPF/1(In1)
  3vector LPF/1(Out1) -> Sum/1

== system AttitudeComplementary/Accel Comp/Subsystem/RB2LTP ==
  Euler : Inport
  11 : Fcn  Expr=cos(u[3])*cos(u[2])
  12 : Fcn  Expr=sin(u[3])*cos(u[2])
  13 : Fcn  Expr=-sin(u[2])
  21 : Fcn  Expr=cos(u[3])*sin(u[2])*sin(u[1])-sin(u[3])*cos(u[1])
  22 : Fcn  Expr=sin(u[3])*sin(u[2])*sin(u[1])+cos(u[3])*cos(u[1])
  23 : Fcn  Expr=cos(u[2])*sin(u[1])
  31 : Fcn  Expr=cos(u[3])*sin(u[2])*cos(u[1])+sin(u[3])*sin(u[1])
  32 : Fcn  Expr=sin(u[3])*sin(u[2])*cos(u[1])-cos(u[3])*sin(u[1])
  33 : Fcn  Expr=cos(u[2])*cos(u[1])
  Mux2 : Mux  Inputs=9
  Reshape : Reshape  OutputDimensionality=Customize  OutputDimensions=[3,3]
  Rot : Outport
  wires:
  33/1 -> Mux2/9
  32/1 -> Mux2/8
  31/1 -> Mux2/7
  23/1 -> Mux2/6
  22/1 -> Mux2/5
  21/1 -> Mux2/4
  13/1 -> Mux2/3
  12/1 -> Mux2/2
  11/1 -> Mux2/1
  Mux2/1 -> Reshape/1
  Euler/1 -> 11/1, 33/1, 32/1, 31/1, 23/1, 22/1, 21/1, 13/1, 12/1
  Reshape/1 -> Rot/1

== system AttitudeComplementary/Accel Comp/get Centripetal/3vector LPF ==
  In1 : Inport  Orientation=left
  Demux : Demux  Orientation=left  Outputs=3
  Low Pass1 : Subsystem  Orientation=left  mask(DiscretizedZeroPole){Zeros=[], Poles=[-flpf], Gain=flpf, AbsTol=auto, SampleTime=SampleT, method=tustin, Wc=1}
      mask prompts: Zeros "Zeros (enter in s-main:)"; Poles "Poles (enter in s-domain:)"; Gain "Gain (enter in s-domain:)"; AbsTol "Absolute tolerance:"; SampleTime "Sample time:"; Wc "Critical Frequency (Hz):"
      mask help: Continuous mask uses c2d to transform parameters onto the Discrete Zero-Pole block inside.
      mask init:
      | st=SampleTime;
      | if length(st)>1
      |     st=SampleTime(1);
      | end
      | if(st>0)
      |     [zerosd,polesd,gaind] = sldiscutil('disczpk', {st,method,Wc,Zeros,Poles,Gain});
      | end	
      | s = get_param(gcb,'maskvalues');
      | zeross = s{1};
      | poless = s{2};
      | gainss = s{3};
      | %zerosc = eval(zeross);
      | %polesc = eval(poless);
      | %gainsc = eval(gainss);
      | sldiscutil('initzpkmask', st);
      | if(st==0)
      | set_param([gcb '/Zero Pole'], 'AbsoluteTolerance', AbsTol);
      | end
      mask StyleString: edit,edit,edit,edit,edit,popup(zoh|foh|tustin|prewarp|matched),edit
      mask CallbackString: |||||hidecrit|
      mask Display:
      | droots(zeross,poless,gainss)
      | text( 0.5, 1.0, method, 'verticalAlignment','top')
  Low Pass2 : Subsystem  Orientation=left  mask(DiscretizedZeroPole){Zeros=[], Poles=[-flpf], Gain=flpf, AbsTol=auto, SampleTime=SampleT, method=tustin, Wc=1}
      mask prompts: Zeros "Zeros (enter in s-main:)"; Poles "Poles (enter in s-domain:)"; Gain "Gain (enter in s-domain:)"; AbsTol "Absolute tolerance:"; SampleTime "Sample time:"; Wc "Critical Frequency (Hz):"
      mask help: Continuous mask uses c2d to transform parameters onto the Discrete Zero-Pole block inside.
      mask init: same as AttitudeComplementary/Accel Comp/get Centripetal/3vector LPF/Low Pass1
      mask StyleString: edit,edit,edit,edit,edit,popup(zoh|foh|tustin|prewarp|matched),edit
      mask CallbackString: |||||hidecrit|
      mask Display:
      | droots(zeross,poless,gainss)
      | text( 0.5, 1.0, method, 'verticalAlignment','top')
  Low Pass3 : Subsystem  Orientation=left  mask(DiscretizedZeroPole){Zeros=[], Poles=[-flpf], Gain=flpf, AbsTol=auto, SampleTime=SampleT, method=tustin, Wc=1}
      mask prompts: Zeros "Zeros (enter in s-main:)"; Poles "Poles (enter in s-domain:)"; Gain "Gain (enter in s-domain:)"; AbsTol "Absolute tolerance:"; SampleTime "Sample time:"; Wc "Critical Frequency (Hz):"
      mask help: Continuous mask uses c2d to transform parameters onto the Discrete Zero-Pole block inside.
      mask init: same as AttitudeComplementary/Accel Comp/get Centripetal/3vector LPF/Low Pass1
      mask StyleString: edit,edit,edit,edit,edit,popup(zoh|foh|tustin|prewarp|matched),edit
      mask CallbackString: |||||hidecrit|
      mask Display:
      | droots(zeross,poless,gainss)
      | text( 0.5, 1.0, method, 'verticalAlignment','top')
  Mux : Mux  Orientation=left  Inputs=3
  Out1 : Outport  Orientation=left
  wires:
  Demux/1 -> Low Pass1/1(In1)
  Demux/2 -> Low Pass2/1(In1)
  Demux/3 -> Low Pass3/1(In1)
  Low Pass1/1(Out1) -> Mux/1
  Low Pass2/1(Out1) -> Mux/2
  Low Pass3/1(Out1) -> Mux/3
  In1/1 -> Demux/1
  Mux/1 -> Out1/1

== system AttitudeComplementary/Get GPS in LTP/Geod2LTP2/ECEF2LTP (UEN) ==
  ECEF coordinates : Inport
  "Long, Lat" : Inport  Port=2
  Deg2R : Gain  Gain=pi/180  SaturateOnIntegerOverflow=on
  Demux3 : Demux  Outputs=2
  From Body to Universal1 : Subsystem
  Product1 : Product  Multiplication=Matrix(*)  SaturateOnIntegerOverflow=on  InputSameDT=on
  Out : Outport
  wires:
  "Long, Lat"/1 -> Deg2R/1
  Product1/1 -> Out/1
  Demux3/2 -> From Body to Universal1/2(lat)
  Demux3/1 -> From Body to Universal1/1(long)
  Deg2R/1 -> Demux3/1
  ECEF coordinates/1 -> Product1/2
  From Body to Universal1/1(DCM) -> Product1/1

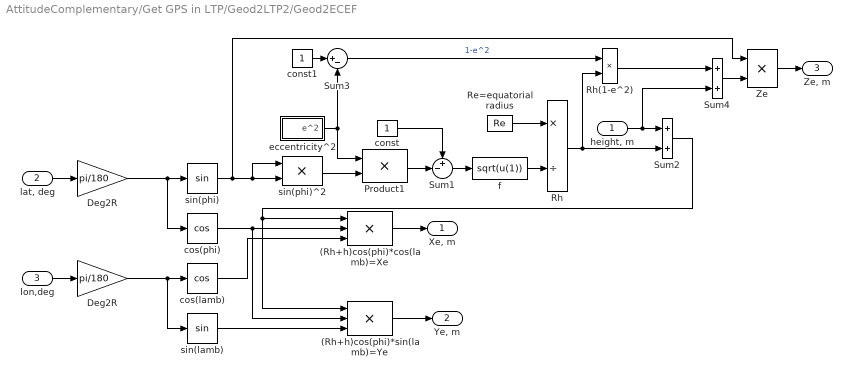
== system AttitudeComplementary/Get GPS in LTP/Geod2LTP2/Geod2ECEF ==
  "height, m" : Inport
  "lat, deg" : Inport  Port=2
  lon,deg : Inport  Port=3
  (Rh+h)cos(phi)*cos(lamb)=Xe : Product  Inputs=3  SaturateOnIntegerOverflow=on  InputSameDT=on
  (Rh+h)cos(phi)*sin(lamb)=Ye : Product  Inputs=3  SaturateOnIntegerOverflow=on  InputSameDT=on
  Deg2R : Gain  Gain=pi/180  SaturateOnIntegerOverflow=on
  "Deg2R " : Gain  Gain=pi/180  SaturateOnIntegerOverflow=on
  Product1 : Product  SaturateOnIntegerOverflow=on  InputSameDT=on
  Re=equatorial radius : Constant  Value=Re
  Rh : Product  Inputs=*/  SaturateOnIntegerOverflow=on  InputSameDT=on
  Rh(1-e^2) : Product  SaturateOnIntegerOverflow=on  InputSameDT=on
  Sum1 : Sum  Inputs=+-|  SaturateOnIntegerOverflow=on  InputSameDT=on
  Sum2 : Sum  SaturateOnIntegerOverflow=on  InputSameDT=on
      settings: AttributesFormatString=Rh+h
  Sum3 : Sum  Inputs=|+-  SaturateOnIntegerOverflow=on  InputSameDT=on
  Sum4 : Sum  SaturateOnIntegerOverflow=on  InputSameDT=on
      settings: AttributesFormatString=(1-e^2)Rh+h
  Ze : Product  SaturateOnIntegerOverflow=on  InputSameDT=on
  const : Constant
  const1 : Constant
  cos(lamb) : Trigonometry  Operator=cos
  cos(phi) : Trigonometry  Operator=cos
  eccentricity^2 : Subsystem
  f : Fcn  Expr=sqrt(u(1))
  sin(lamb) : Trigonometry
  sin(phi) : Trigonometry
  sin(phi)^2 : Product  SaturateOnIntegerOverflow=on  InputSameDT=on
  "Xe, m " : Outport
  "Ye, m " : Outport  Port=2
  "Ze, m " : Outport  Port=3
  wires:
  "lat, deg"/1 -> Deg2R/1
  sin(phi)/1 -> sin(phi)^2/1, sin(phi)^2/2, Ze/1
  f/1 -> Rh/2
  Re=equatorial radius/1 -> Rh/1
  Rh/1 -> Sum2/2, Rh(1-e^2)/2
  Product1/1 -> Sum1/2
  Sum1/1 -> f/1
  const/1 -> Sum1/1
  "height, m"/1 -> Sum4/2, Sum2/1
  eccentricity^2/1(e^2) -> Product1/1, Sum3/2
  sin(phi)^2/1 -> Product1/2
  const1/1 -> Sum3/1
  Sum3/1 -> Rh(1-e^2)/1  "1-e^2"
  Rh(1-e^2)/1 -> Sum4/1
  Sum4/1 -> Ze/2
  lon,deg/1 -> "Deg2R "/1
  cos(phi)/1 -> (Rh+h)cos(phi)*cos(lamb)=Xe/2, (Rh+h)cos(phi)*sin(lamb)=Ye/2
  cos(lamb)/1 -> (Rh+h)cos(phi)*cos(lamb)=Xe/3
  sin(lamb)/1 -> (Rh+h)cos(phi)*sin(lamb)=Ye/3
  Ze/1 -> "Ze, m "/1
  Deg2R/1 -> cos(phi)/1, sin(phi)/1
  "Deg2R "/1 -> cos(lamb)/1, sin(lamb)/1
  Sum2/1 -> (Rh+h)cos(phi)*sin(lamb)=Ye/1, (Rh+h)cos(phi)*cos(lamb)=Xe/1
  (Rh+h)cos(phi)*cos(lamb)=Xe/1 -> "Xe, m "/1
  (Rh+h)cos(phi)*sin(lamb)=Ye/1 -> "Ye, m "/1

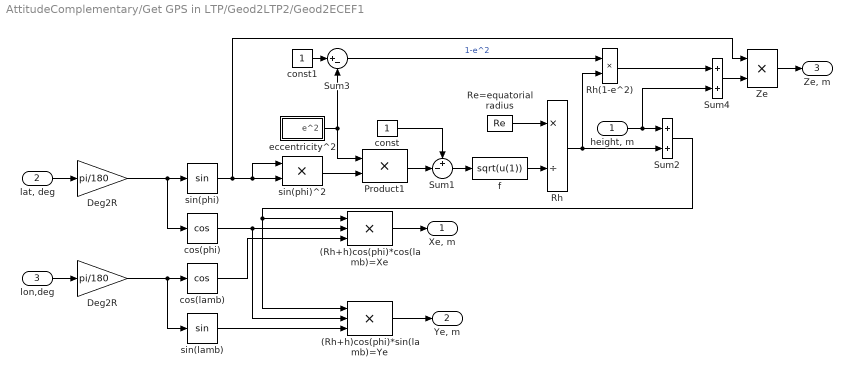
== system AttitudeComplementary/Get GPS in LTP/Geod2LTP2/Geod2ECEF1 ==
  "height, m" : Inport
  "lat, deg" : Inport  Port=2
  lon,deg : Inport  Port=3
  (Rh+h)cos(phi)*cos(lamb)=Xe : Product  Inputs=3  SaturateOnIntegerOverflow=on  InputSameDT=on
  (Rh+h)cos(phi)*sin(lamb)=Ye : Product  Inputs=3  SaturateOnIntegerOverflow=on  InputSameDT=on
  Deg2R : Gain  Gain=pi/180  SaturateOnIntegerOverflow=on
  "Deg2R " : Gain  Gain=pi/180  SaturateOnIntegerOverflow=on
  Product1 : Product  SaturateOnIntegerOverflow=on  InputSameDT=on
  Re=equatorial radius : Constant  Value=Re
  Rh : Product  Inputs=*/  SaturateOnIntegerOverflow=on  InputSameDT=on
  Rh(1-e^2) : Product  SaturateOnIntegerOverflow=on  InputSameDT=on
  Sum1 : Sum  Inputs=+-|  SaturateOnIntegerOverflow=on  InputSameDT=on
  Sum2 : Sum  SaturateOnIntegerOverflow=on  InputSameDT=on
      settings: AttributesFormatString=Rh+h
  Sum3 : Sum  Inputs=|+-  SaturateOnIntegerOverflow=on  InputSameDT=on
  Sum4 : Sum  SaturateOnIntegerOverflow=on  InputSameDT=on
      settings: AttributesFormatString=(1-e^2)Rh+h
  Ze : Product  SaturateOnIntegerOverflow=on  InputSameDT=on
  const : Constant
  const1 : Constant
  cos(lamb) : Trigonometry  Operator=cos
  cos(phi) : Trigonometry  Operator=cos
  eccentricity^2 : Subsystem
  f : Fcn  Expr=sqrt(u(1))
  sin(lamb) : Trigonometry
  sin(phi) : Trigonometry
  sin(phi)^2 : Product  SaturateOnIntegerOverflow=on  InputSameDT=on
  "Xe, m " : Outport
  "Ye, m " : Outport  Port=2
  "Ze, m " : Outport  Port=3
  wires:
  (Rh+h)cos(phi)*sin(lamb)=Ye/1 -> "Ye, m "/1
  (Rh+h)cos(phi)*cos(lamb)=Xe/1 -> "Xe, m "/1
  Sum2/1 -> (Rh+h)cos(phi)*cos(lamb)=Xe/1, (Rh+h)cos(phi)*sin(lamb)=Ye/1
  "Deg2R "/1 -> sin(lamb)/1, cos(lamb)/1
  Deg2R/1 -> sin(phi)/1, cos(phi)/1
  Ze/1 -> "Ze, m "/1
  sin(lamb)/1 -> (Rh+h)cos(phi)*sin(lamb)=Ye/3
  cos(lamb)/1 -> (Rh+h)cos(phi)*cos(lamb)=Xe/3
  cos(phi)/1 -> (Rh+h)cos(phi)*sin(lamb)=Ye/2, (Rh+h)cos(phi)*cos(lamb)=Xe/2
  lon,deg/1 -> "Deg2R "/1
  Sum4/1 -> Ze/2
  Rh(1-e^2)/1 -> Sum4/1
  Sum3/1 -> Rh(1-e^2)/1  "1-e^2"
  const1/1 -> Sum3/1
  sin(phi)^2/1 -> Product1/2
  eccentricity^2/1(e^2) -> Sum3/2, Product1/1
  "height, m"/1 -> Sum2/1, Sum4/2
  const/1 -> Sum1/1
  Sum1/1 -> f/1
  Product1/1 -> Sum1/2
  Rh/1 -> Rh(1-e^2)/2, Sum2/2
  Re=equatorial radius/1 -> Rh/1
  f/1 -> Rh/2
  sin(phi)/1 -> Ze/1, sin(phi)^2/2, sin(phi)^2/1
  "lat, deg"/1 -> Deg2R/1

== system AttitudeComplementary/Plant Model/Plant/6-DOF EOM ==
  "[F,M]" : Inport
  Vb Corr : Inport  Orientation=left  Port=2
  Angular Rates : Integrator  InitialCondition=PQR_0'
  Demux1 : Demux  Outputs=[3 3]
  Euler Angles : Integrator  InitialCondition=Euler_0'
  Get Euler Dot : Subsystem
      mask Display:
      | port_label('input', 1, 'p, q, r')
      | port_label('input', 2, 'Euler')
      | port_label('output', 1, 'Euler_dot')
  Mux : Mux  Orientation=left  Inputs=[3;3]
  NED2NEU : Gain  Gain=[1 0 0;0 1 0;0 0 -1]  Multiplication=Matrix(K*u)  SaturateOnIntegerOverflow=on
  Position : Integrator  InitialCondition=Pos_0'
  RB2L * Vb : Product  Multiplication=Matrix(*)  SaturateOnIntegerOverflow=on  InputSameDT=on
  RB2LTP : Subsystem
  Velocities Body : Integrator  InitialCondition=Vb_0'
  "[V1,2,3,W1,2,3]" : Subsystem
  X,Y,Z (LTP) : Outport
  "Vx, Vy, Vz" : Outport  Port=2
  Euler : Outport  Port=3
  "p, q, r" : Outport  Orientation=left  Port=4
  Euler_dot : Outport  Port=5
  Vb : Outport  Port=6
  Ab : Outport  Port=7
  Ab meas : Outport  Port=8
  wires:
  "[V1,2,3,W1,2,3]"/1("Acc_meas ") -> Ab meas/1
  Euler Angles/1 -> "[V1,2,3,W1,2,3]"/2(Euler), Get Euler Dot/2(Euler), Euler/1, RB2LTP/1(Euler)
  Demux1/1 -> Ab/1, Velocities Body/1
  "[V1,2,3,W1,2,3]"/2(V*dot) -> Demux1/1
  Demux1/2 -> Angular Rates/1
  "[F,M]"/1 -> "[V1,2,3,W1,2,3]"/1("[F ; M]")
  RB2LTP/1(Rot) -> RB2L * Vb/1
  Velocities Body/1 -> Vb/1, RB2L * Vb/2
  Mux/1 -> "[V1,2,3,W1,2,3]"/3(V*)
  Position/1 -> X,Y,Z (LTP)/1
  Angular Rates/1 -> Get Euler Dot/1(p,q,r), Mux/2, "p, q, r"/1
  RB2L * Vb/1 -> NED2NEU/1, "Vx, Vy, Vz"/1  "NED"
  NED2NEU/1 -> Position/1
  Get Euler Dot/1(Euler_dot) -> Euler Angles/1, Euler_dot/1
  Vb Corr/1 -> Mux/1

== system AttitudeComplementary/Plant Model/Plant/Engine Model ==
  dt : Inport
  Vmag : Inport  Port=2
  Constant4 : Constant  Value=0
  Get To1 : Subsystem
  Mux : Mux  Inputs=2
  Mux1 : Mux  Inputs=3
  Thrust Available (lbs) : Fcn  Expr=u(1) - 0.047*sqrt(u(1))*u(2)
  kg2N : Gain  Gain=ISA_g  SaturateOnIntegerOverflow=on
  lbs2kg : Gain  Gain=0.45359237  SaturateOnIntegerOverflow=on
  RPM : Outport
  Thrust : Outport  Port=2
  wires:
  Get To1/1(RPM) -> RPM/1
  dt/1 -> Get To1/1(dt)
  Get To1/2(To) -> Mux/1
  Mux/1 -> Thrust Available (lbs)/1
  Thrust Available (lbs)/1 -> lbs2kg/1
  Vmag/1 -> Mux/2
  Mux1/1 -> Thrust/1
  lbs2kg/1 -> kg2N/1
  Constant4/1 -> Mux1/2, Mux1/3
  kg2N/1 -> Mux1/1

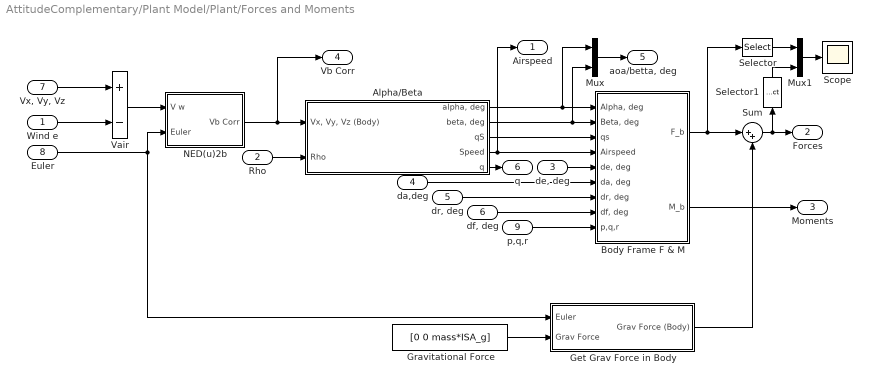
== system AttitudeComplementary/Plant Model/Plant/Forces and Moments ==
  Wind e : Inport
  Rho : Inport  Port=2
  "de, deg" : Inport  Port=3
  da,deg : Inport  Port=4
  "dr, deg" : Inport  Port=5
  "df, deg" : Inport  Port=6
  "Vx, Vy, Vz " : Inport  Port=7
  Euler : Inport  Port=8  PortDimensions=3
  p,q,r : Inport  Port=9
  Alpha/Beta : Subsystem
  Body Frame F & M : Subsystem
  Get Grav Force in Body : Subsystem
  Gravitational Force : Constant  Value=[0 0 mass*ISA_g]  VectorParams1D=off
  Mux : Mux  Inputs=2
  Mux1 : Mux  Inputs=2
  NED(u)2b : Subsystem
  Scope : Scope
      settings: SaveName=ScopeData5
  Selector : Selector  IndexOptions=Index vector (dialog)  Indices=3  OutputSizes=1  InputPortWidth=3
  Selector1 : Selector  Orientation=up  IndexOptions=Index vector (dialog)  Indices=3  OutputSizes=1  InputPortWidth=3
  Sum : Sum  Inputs=|++  SaturateOnIntegerOverflow=on
  Vair : Sum  Inputs=+-  SaturateOnIntegerOverflow=on  InputSameDT=on
  Airspeed : Outport
  Forces : Outport  Port=2
  Moments : Outport  Port=3
  Vb Corr : Outport  Port=4
  "aoa/betta, deg" : Outport  Port=5
  q : Outport  Port=6
  wires:
  Get Grav Force in Body/1(Grav Force (Body)) -> Sum/2
  Selector1/1 -> Mux1/2
  Mux1/1 -> Scope/1
  Selector/1 -> Mux1/1
  Mux/1 -> "aoa/betta, deg"/1
  Alpha/Beta/5(q) -> q/1
  "Vx, Vy, Vz "/1 -> Vair/1
  Vair/1 -> NED(u)2b/1(V w)
  Euler/1 -> NED(u)2b/2(Euler), Get Grav Force in Body/1(Euler)
  Rho/1 -> Alpha/Beta/2(Rho)
  NED(u)2b/1(Vb Corr) -> Alpha/Beta/1("Vx, Vy, Vz (Body)"), Vb Corr/1
  Body Frame F & M/2(M_b) -> Moments/1
  Gravitational Force/1 -> Get Grav Force in Body/2(Grav Force)
  Body Frame F & M/1(F_b) -> Selector/1, Sum/1
  Sum/1 -> Selector1/1, Forces/1
  Alpha/Beta/3(qS) -> Body Frame F & M/3(qs)
  Alpha/Beta/4(Speed) -> Body Frame F & M/4(Airspeed), Airspeed/1
  "df, deg"/1 -> Body Frame F & M/8("df, deg")
  p,q,r/1 -> Body Frame F & M/9(p,q,r)
  Alpha/Beta/2("beta, deg") -> Mux/2, Body Frame F & M/2("Beta, deg")
  "dr, deg"/1 -> Body Frame F & M/7("dr, deg")
  da,deg/1 -> Body Frame F & M/6("da, deg")
  Alpha/Beta/1("alpha, deg") -> Mux/1, Body Frame F & M/1("Alpha, deg")
  "de, deg"/1 -> Body Frame F & M/5("de, deg")
  Wind e/1 -> Vair/2

== system AttitudeComplementary/Plant Model/Plant/Get GPS ==
  XYZ (NEU) : Inport
  Angle Conversion : aerolibconvert2/Angle Conversion  SystemSampleTime=-1  IU=deg  OU=rad
  Demux : Demux  Outputs=6
  Demux2 : Demux  Outputs=2
  Flat Earth to LLA : aerolibtransform2/Flat Earth to LLA  SystemSampleTime=-1  units=Metric (MKS)  ptype=Earth (WGS84)  F=1/298.257223563  R=6378137  LL0=[37.0004768371582, -122.061897277832]  psi=0
  MATLAB Fcn : MATLABFcn  MATLABFcn=u(1)*clock  OutputSignalType=real
  NEU2NED : Gain  Gain=[1 0 0;0 1 0;0 0 -1]  Multiplication=Matrix(K*u)  SaturateOnIntegerOverflow=on
  Rounding Function : Rounding
  Zero level trust : Constant  Value=0
  Zero level trust1 : Constant
  Zero level trust2 : Constant  Value=0
  GPS Month : Outport
  GPS Day : Outport  Port=2
  GPS Year : Outport  Port=3
  GPS Hr : Outport  Port=4
  GPS Min : Outport  Port=5
  GPS Sec : Outport  Port=6
  GPS Frac Sec : Outport  Port=7
  GPS Lat (rad) : Outport  Port=8
  GPS Long (rad) : Outport  Port=9
  GPS H (m) : Outport  Port=10
  wires:
  NEU2NED/1 -> Flat Earth to LLA/1
  Zero level trust/1 -> Flat Earth to LLA/2
  XYZ (NEU)/1 -> NEU2NED/1
  Flat Earth to LLA/1 -> Angle Conversion/1
  Flat Earth to LLA/2 -> GPS H (m)/1
  Zero level trust1/1 -> MATLAB Fcn/1
  MATLAB Fcn/1 -> Demux/1
  Demux/2 -> GPS Month/1
  Demux/3 -> GPS Day/1
  Demux/1 -> GPS Year/1
  Demux/4 -> GPS Hr/1
  Demux/5 -> GPS Min/1
  Demux/6 -> Rounding Function/1
  Rounding Function/1 -> GPS Sec/1
  Zero level trust2/1 -> GPS Frac Sec/1
  Angle Conversion/1 -> Demux2/1
  Demux2/1 -> GPS Lat (rad)/1
  Demux2/2 -> GPS Long (rad)/1

== system AttitudeComplementary/Plant Model/Plant/ISA Atmosphere & Winds ==
  "X, Y, Z" : Inport
  Correct Wind : Constant  Value=[0;0;0]
  Get Z : Selector  IndexOptions=Index vector (dialog)  Indices=[3]  OutputSizes=[(-2)]  InputPortWidth=3
  ISA Atmosphere Model1 : aerolibatmos2/ISA Atmosphere Model  SystemSampleTime=-1  custom=off  g=9.80665  gamma=1.4  R=287.0531  L=0.0065  h_trop=11000  h_strat=20000  rho0=1.225  P0=101325  T0=288.15
  Terminator : Terminator
  Terminator1 : Terminator
  Rho : Outport
  Wind : Outport  Port=2
  AirPressure (Pa) : Outport  Port=3
  wires:
  "X, Y, Z"/1 -> Get Z/1
  Get Z/1 -> ISA Atmosphere Model1/1
  ISA Atmosphere Model1/4 -> Rho/1
  ISA Atmosphere Model1/1 -> Terminator/1
  ISA Atmosphere Model1/2 -> Terminator1/1
  ISA Atmosphere Model1/3 -> AirPressure (Pa)/1
  Correct Wind/1 -> Wind/1
